simulink model "example_ModelDoc"  (R2018b)
settings: Solver=ode45  StartTime=0.0  StopTime=10  RelTol=1e-3
undefined symbols (not defined in the file): path_carnot
libraries: carnot x8
settings Model: Creator=goettsche  LastModifiedBy=drhf
settings DataIOCC: LimitDataPoints=on  SaveFormat=Array  SignalLoggingSaveFormat=ModelDataLogs  ReturnWorkspaceOutputs=on
settings OptimizationCC: LifeSpan=inf
settings DebuggingCC: ReadBeforeWriteMsg=DisableAll  WriteAfterWriteMsg=DisableAll  WriteAfterReadMsg=DisableAll  SaveWithParameterizedLinksMsg=none  UnderspecifiedInitializationDetection=Classic  MergeDetectMultiDrivingBlocksExec=none  MultiTaskDSMMsg=none  MultiTaskCondExecSysMsg=none  SFUnexpectedBacktrackingDiag=warning  SFNoUnconditionalDefaultTransitionDiag=warning  SFExecutionAtInitializationDiag=none
settings HardwareCC: ProdBitPerPointer=32  ProdBitPerSizeT=32  ProdBitPerPtrDiffT=32  ProdLargestAtomicFloat=None  ProdIntDivRoundTo=Undefined  ProdEndianess=Unspecified  ProdWordSize=32  ProdHWDeviceType=32-bit Generic  TargetUnknown=on
settings ModelReferenceCC: UpdateModelReferenceTargets=IfOutOfDate  PropagateSignalLabelsOutOfModel=off
settings SFSimCC: SFSimEcho=off  SimUseLocalCustomCode=off
settings RTWCC: RTWUseLocalCustomCode=off
settings CodeAppCC: StateflowObjectComments=on
settings GRTTargetCC: TargetLangStandard=C89/C90 (ANSI)  GeneratePreprocessorConditionals=Disable all
settings ConfigComp: CovMetricSettings=dw  CovHtmlReporting=on  CovSaveCumulativeToWorkspaceVar=on  CovSaveSingleToWorkspaceVar=on  CovExternalEMLEnable=off

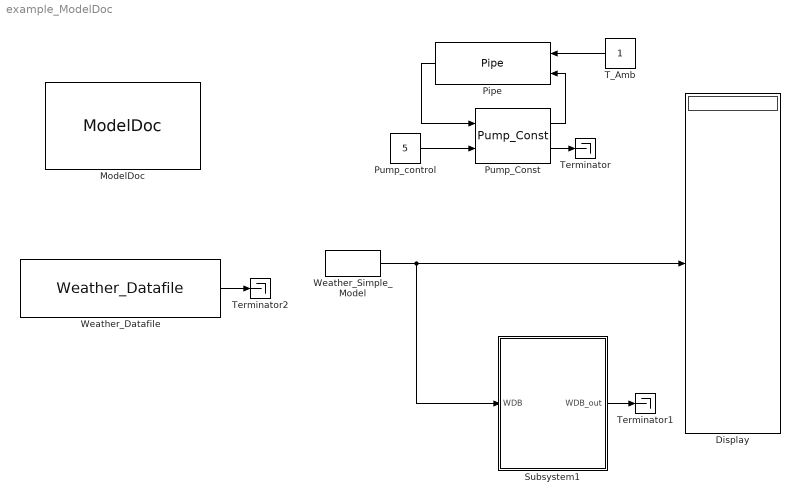
== system example_ModelDoc ==
  " ModelDoc" : carnot/Toolbox/ModelDoc  SystemSampleTime=-1
      settings: SourceProductName=Carnot
  Display : Display
  Pipe : carnot/Hydraulics/Pipe  dia=0.02  len=10  hgt=5  uloss=100/20/10  cond=0  cwall=1000  t0=20  lin=100/0.2  qua=100/0.2^2  nodes=10
      settings: SourceProductName=Carnot
  Pump_Const : carnot/Hydraulics/Pump_Const  mdotmax=1200/3600  dia=0.0157  p0=3e5  fluid_id=Water  mix=0  mix2=0  mix3=0  UA=3  mcp=4000  Tini=20  e0=10  e1=10  e2=-1
      settings: SourceProductName=Carnot
  Pump_control : Constant  Value=5
  Subsystem1 : Subsystem  TreatAsAtomicUnit=on
  T_Amb : Constant
  Terminator : Terminator
  Terminator1 : Terminator
  Terminator2 : Terminator
  Weather_Datafile : carnot/Weather/Weather_Datafile  PathName=path_carnot('data')  FileName='DE_TRY2010_04_averageYear.mat'  UserParam=off  VariableName=DE_TRY2010_04_averageYear  SampleTime=3600
      settings: SourceProductName=Carnot
  Weather_Simple_Model : carnot/Weather/Weather_Simple_Model  Ibn=900  Idg=100  tamb=5  deltaTsky=-6  rh=50  precip="10e-3/24/3600           % 10 mm in 24 h"  cloud=0.125  p=1013e2  vw=1  wdir=270  lat=60  colangle=0  colazi=0  colrot=0
      settings: SourceProductName=Carnot
  wires:
  Weather_Simple_Model/1 -> Subsystem1/1(WDB), Display/1
  Pump_control/1 -> Pump_Const/2
  Pump_Const/1 -> Pipe/2
  Pipe/1 -> Pump_Const/1
  T_Amb/1 -> Pipe/1
  Pump_Const/2 -> Terminator/1
  Subsystem1/1(WDB_out) -> Terminator1/1
  Weather_Datafile/1 -> Terminator2/1

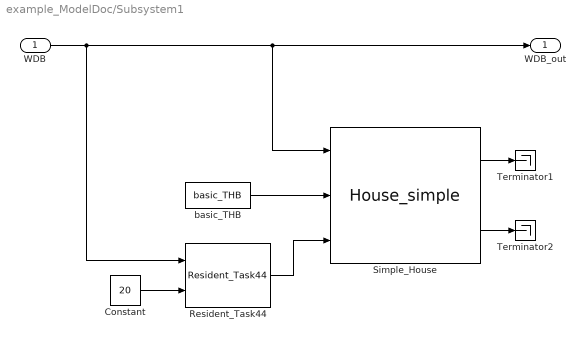
== system example_ModelDoc/Subsystem1 ==
  WDB : Inport
  Constant : Constant  Value=20
  Resident_Task44 : carnot/Load/Houses/Resident_Task44  period=24*3600  rep_seq_te=[0 1 6 7 8 9 11 12 13 18 19 20 22 23]*3600  rep_seq_de=[1 5 1 1 1 2 1 1 4 2 1 2 1 1]*3600  rep_seq_ye=[105 55 392.5 457.5 420 55 250 55 120 170 615 420 442.5 355]  rep_seq_to=[0 6 7 8 9 11 12 13 14 15 17 18 20 21 22]*3600  rep_seq_do=[6 1 1 1 2 1 1 1 1 2 1 2 1 1 2]*3600  rep_seq_yo=[4 2 3 2 0 1 3 2 1 0 1 2 4 3 4]*60  Topen=24  Tclose=23  TrAboveTa=2  TaTooCold=12  timeFIR=24  TaIni=12  starttime=8  stoptime=22  TroomShadeOn=23.8  TroomShadeOff=22.8  SolarShadeOn=300  SolarShadeOff=200  max_shade=1  CalcAirComp=off  mdotCO2=0  mdotH2O=0  mdotVOC=0
      settings: SourceProductName=Carnot
  Simple_House : carnot/Load/Houses/House_simple  tini=20  dtroom=inf  Tmeaninside=23.8  deltathetai=3.8  Tmeanoutside=11  deltathetae=9.3  tshift=319*3600  PathName=fullfile(path_carnot('libsl'), 'Load', 'Houses', 'House_simple', 'parameter_set')  FileName='Default_HouseSimple.mat'  userPath=off  userParam=off  Ahabit=140  Hroom=2.5  slabwidth=10  slablength=7  dwall=0.4  UAwall=100  capa=500000  utot=0.183  gammat=0  cond_ground=2  cp_ground=800  rho_ground=2500  Awindow=[12 4 3 4]  AziWin=[0 90 -180 -90]  Uwindow=[2 2 2 2]  Gwindow=[0.5 0.5 0.5 0.5]  alpha=10  H=1.2  W=1  Nwin=4  Ventilationrate=0.4  Heatrecovery=0  pnom=10000  dtnom=49.83  expo=1.3  mcap=10*4812  lin=100  qua=100
      settings: SourceProductName=Carnot
  Terminator1 : Terminator
  Terminator2 : Terminator
  basic_THB : carnot/Basic/Hydraulics/basic_THB  t=10  mdot=100/3600  p=2e5  ID=Pressure Drop from Massflow  fluid=Water  mix=0  mix2=0  mix3=0  dia=.03  hgt=1
      settings: SourceProductName=Carnot
  WDB_out : Outport
  wires:
  WDB/1 -> Resident_Task44/1, Simple_House/1, WDB_out/1
  basic_THB/1 -> Simple_House/2
  Simple_House/1 -> Terminator1/1
  Simple_House/2 -> Terminator2/1
  Resident_Task44/1 -> Simple_House/3
  Constant/1 -> Resident_Task44/2
